simulink model "Task2_Fault_Mag1"  (R2023a)
settings: Solver=ode5  StartTime=0.0  StopTime=15  FixedStep=0.025  RelTol=1e-3  EnableMultiTasking=on
libraries: simulink x3
settings Model: Creator=Guptas  LastModifiedBy=Guptas
settings DataIOCC: LimitDataPoints=on  SaveFormat=Array  SignalLoggingSaveFormat=ModelDataLogs  ReturnWorkspaceOutputs=off  SignalLoggingName=sigsOut
settings OptimizationCC: BlockReduction=off  BooleanDataType=off
settings DebuggingCC: SaveWithParameterizedLinksMsg=none  UnderspecifiedInitializationDetection=Classic  MergeDetectMultiDrivingBlocksExec=none  SignalResolutionControl=TryResolveAllWithWarning  MultiTaskDSMMsg=warning  MultiTaskCondExecSysMsg=none  UnconnectedInputMsg=warning  UnconnectedOutputMsg=warning  UnconnectedLineMsg=warning
settings HardwareCC: ProdBitPerPointer=32  ProdBitPerSizeT=32  ProdBitPerPtrDiffT=32  ProdLargestAtomicFloat=None  ProdIntDivRoundTo=Undefined  ProdEndianess=Unspecified  ProdWordSize=32  ProdHWDeviceType=32-bit Generic  TargetUnknown=on
settings ModelReferenceCC: PropagateSignalLabelsOutOfModel=off
settings GRTTargetCC: CombineOutputUpdateFcns=off  GRTInterface=on
settings ConfigComp: CovMetricSettings=dw  CovSaveCumulativeToWorkspaceVar=on  CovSaveSingleToWorkspaceVar=on

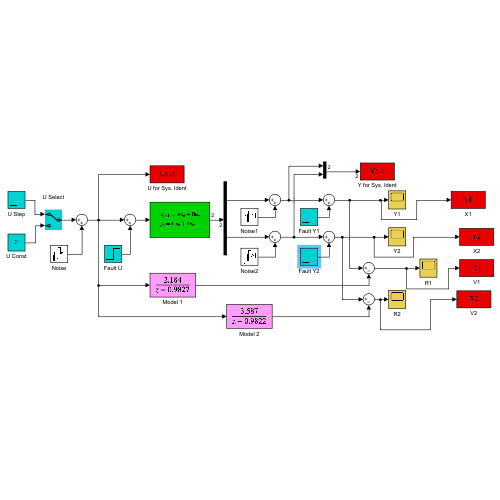
[thumbnail: Simulink's stored preview of the top-level diagram]
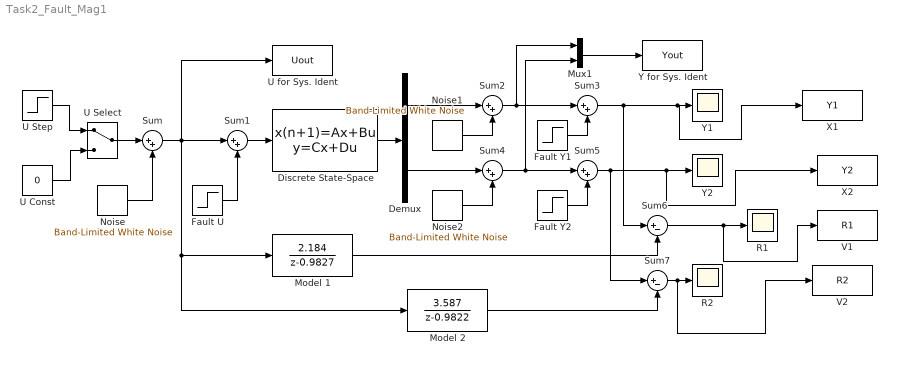
== system Task2_Fault_Mag1 ==
  Demux : Demux  Outputs=2
      settings: DisplayOption=none
  Discrete State-Space : DiscreteStateSpace  A=|  B=|  C=[1 0; 0 1]  D=[0;0]  SampleTime=0.025
      A=|
      | [0.9769 0.0038;
      | 0.0936 0.9225]
      B=|
      | [2.1521;
      | 3.8186]
  Fault U : Step  Time=3  After=0  SampleTime=0
  Fault Y1 : Step  Time=3  After=3  SampleTime=0
  Fault Y2 : Step  Time=3  After=3  SampleTime=0
  Model 1 : DiscreteTransferFcn  Numerator=[2.184]  Denominator=[1 -0.9827]  SampleTime=0.025
  Model 2 : DiscreteTransferFcn  Numerator=[3.587]  Denominator=[1 -0.9822]  SampleTime=0.025
  Mux1 : Mux  Inputs=2
  Noise : simulink/Sources/Band-Limited White Noise  Cov=[0.01]  Ts=0.025  seed=[23341]
  Noise1 : simulink/Sources/Band-Limited White Noise  Cov=[0.1]  Ts=0.025  seed=[23341]
  Noise2 : simulink/Sources/Band-Limited White Noise  Cov=[0.1]  Ts=0.025  seed=[23341]
  R1 : Scope
  R2 : Scope
  Sum{,1..5} (6 alike) : Sum  Inputs=|++  SaturateOnIntegerOverflow=on
  Sum6 : Sum  Inputs=|+-  SaturateOnIntegerOverflow=on
  Sum7 : Sum  Inputs=|+-  SaturateOnIntegerOverflow=on
  U Const : Constant  Value=0
  "U Select " : ManualSwitch
  U Step : Step  SampleTime=0
  U for Sys. Ident : ToWorkspace  VariableName=Uout  SampleTime=0.025
  V1 : ToWorkspace  VariableName=R1  SampleTime=0.025
  V2 : ToWorkspace  VariableName=R2  SampleTime=0.025
  X1 : ToWorkspace  VariableName=Y1  SampleTime=0.025
  X2 : ToWorkspace  VariableName=Y2  SampleTime=0.025
  Y for Sys. Ident : ToWorkspace  VariableName=Yout  SampleTime=0.025
  Y1 : Scope
  Y2 : Scope
  wires:
  U Const/1 -> "U Select "/2
  U Step/1 -> "U Select "/1
  Mux1/1 -> Y for Sys. Ident/1
  Discrete State-Space/1 -> Demux/1
  Sum/1 -> Sum1/1, Model 1/1, Model 2/1, U for Sys. Ident/1
  Sum1/1 -> Discrete State-Space/1
  "U Select "/1 -> Sum/1
  Sum2/1 -> Sum3/1, Mux1/1
  Sum4/1 -> Sum5/1, Mux1/2
  Sum3/1 -> X1/1, Y1/1, Sum6/1
  Sum5/1 -> X2/1, Y2/1, Sum7/1
  Model 1/1 -> Sum6/2
  Model 2/1 -> Sum7/2
  Sum7/1 -> V2/1, R2/1
  Sum6/1 -> V1/1, R1/1
  Demux/1 -> Sum2/1
  Demux/2 -> Sum4/1
  Fault U/1 -> Sum1/2
  Noise/1 -> Sum/2
  Noise1/1 -> Sum2/2
  Noise2/1 -> Sum4/2
  Fault Y1/1 -> Sum3/2
  Fault Y2/1 -> Sum5/2
